simulink model "OvenMass"  (R2019b)
settings: Solver=VariableStepAuto  StartTime=0.0  StopTime=500  RelTol=1e-3
model workspace (MAT data in the model file):
  Stefan_Boltzmann_constant = 5.6704e-08
  air_density = 1.225
  air_heat_transfer_coefficient = 0.6
  air_volume_cubic_inch = 1152
  air_volume_cubic_meter = 0.0188778989947
  brick_count = 32
  brick_mass = 2.27
  emissivity_mass = 0.7
  mass_length = 0.1
  mass_mass = 1
  set_temperature = Simulink.Parameter
  set_temperature.Value = 1000
  set_temperature.DataType = 'auto'
  set_temperature.Dimensions = [1 1]
  wire_cross_sectional_area = Simulink.Parameter
  wire_cross_sectional_area.Value = 7.07e-06
  wire_cross_sectional_area.DataType = 'auto'
  wire_cross_sectional_area.Dimensions = [1 1]
  wire_length = Simulink.Parameter
  wire_length.Value = 2.44
  wire_length.DataType = 'auto'
  wire_length.Dimensions = [1 1]
  wire_outer_surface_area = 0.04363
  wire_resistivity = Simulink.Parameter
  wire_resistivity.Value = 0.000135
  wire_resistivity.DataType = 'auto'
  wire_resistivity.Dimensions = [1 1]
  wire_specific_heat = Simulink.Parameter
  wire_specific_heat.Value = 300
  wire_specific_heat.DataType = 'auto'
  wire_specific_heat.Dimensions = [1 1]
libraries: fl_lib x17, nesl_utility x5, ee_lib x4, simulink x2, eePwmGenerator x1
settings Model: SimulationMode=rapid-accelerator  Creator=Lenovo  LastModifiedBy=Lenovo
settings SolverCC: AlgebraicLoopSolver=LineSearch

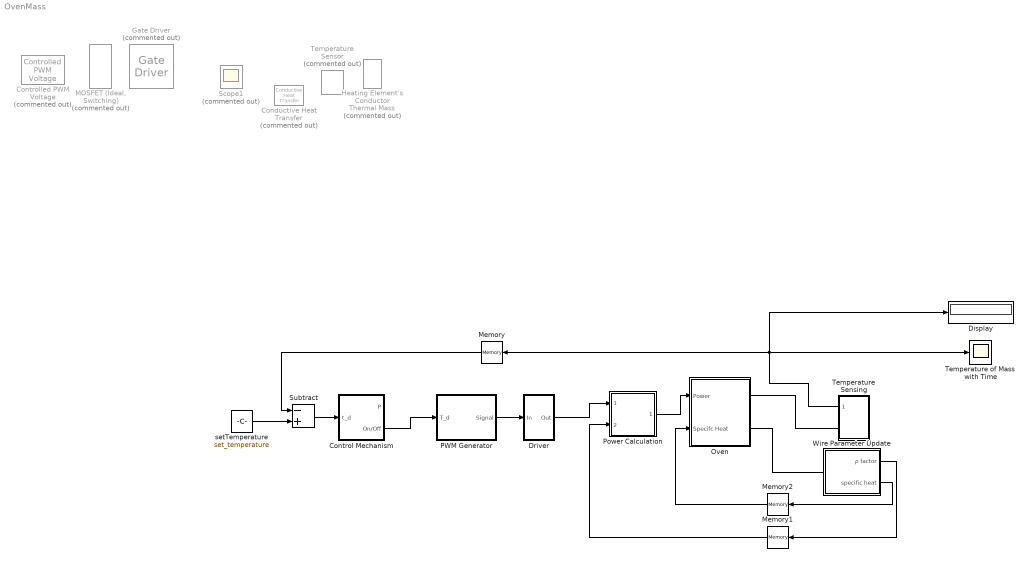
== system OvenMass ==
  Conductive Heat Transfer : fl_lib/Thermal/Thermal Elements/Conductive Heat Transfer  Commented=on  area=1e-4 m^2  thickness=0.1 m  th_cond=401 W/(m*K)  T_specify=off  T_priority=None  T=0 K  T_nominal_specify=off  T_nominal_unit=K  T_nominal_value=1  Q_specify=off  Q_priority=None  Q=0 W  Q_nominal_specify=off  Q_nominal_unit=W  Q_nominal_value=1
      settings: SourceProductName=Simscape
  Control Mechanism : Subsystem
  Controlled PWM Voltage : ee_lib/Integrated Circuits/Controlled PWM Voltage  Commented=on  F=1000 Hz  TD=0 s  pulse_width_offset=0 s  pulse_min=0 s  Vmin=0 V  Vmax=5 V  Vm=5 V  pwm_or_av=1  event_type=1  sample_time=1e-6 s  u_min=0  u_max=1
      settings: SourceProductName=Simscape Electrical  InternalSimscapePortConfiguration="{\"Bottom\":[],\"Left\":[{\"id\":\"u\",\"label\":\"u\",\"type\":\"input\"}],\"Right\":[{\"id\":\"p2\",\"label\":\"PWM\",\"type\":\"foundation.electrical.electrical\"},{\"id\":\"n2\",\"label\":\"REF\",\"type\":\"foundation.electrical.electrical\"}],\"Top\":[]}"
  Display : Display
      settings: Decimation=2
  Driver : Subsystem
  Gate Driver : ee_lib/Semiconductors & Converters/Gate Driver  Commented=on  vHigh=15 V  vLow=0 V  parameterization=1  rHigh=2 Ohm  rLow=2 Ohm  tRise=20 ns  tFall=20 ns  cLoad=10 nF  enable_faults=0  t_fault=1 s  fault_type=1  uHighValue=0.7  uLowValue=0.3  tHigh=50 ns  tLow=50 ns  ZonTime_specify=off  ZonTime_priority=None  ZonTime=0 s  ZoffTime_specify=off  ZoffTime_priority=None  ZoffTime=0 s  uHigh=2.0 V  uLow=0.8 V
      settings: SourceProductName=Simscape Electrical  SourceProductBaseCode=PS  InternalSimscapePortConfiguration="{\"Bottom\":[],\"Left\":[{\"id\":\"u\",\"label\":\"u\",\"type\":\"input\"}],\"Right\":[{\"id\":\"G\",\"label\":\"G\",\"type\":\"foundation.electrical.electrical\"},{\"id\":\"S\",\"label\":\"S\",\"type\":\"foundation.electrical.electrical\"}],\"Top\":[]}"
  Heating Element's Conductor : fl_lib/Thermal/Thermal Elements/Thermal Mass  Commented=on  mass=1 kg  sp_heat=780 J/kg/K  T_specify=off  T_priority=High  T=777 K  T_nominal_specify=off  T_nominal_unit=K  T_nominal_value=1  Q_specify=off  Q_priority=None  Q=0 W  Q_nominal_specify=off  Q_nominal_unit=W  Q_nominal_value=1
  "MOSFET (Ideal, Switching)" : ee_lib/Semiconductors & Converters/MOSFET (Ideal, Switching)  Commented=on  Rds=0.01 Ohm  Goff=1e-6 1/Ohm  Vth=2 V  diode_param=1  diode_Vf=0.8 V  diode_Ron=0.001 Ohm  diode_Goff=1e-5 1/Ohm  diode_C=50e-9 F  diode_iRM=-235 A  diode_iF=300 A  diode_idot=-50 A/us  diode_trr_param=1  diode_trr_factor=3  diode_trr=15 us  diode_Qrr=1500 s*uA  thermal_loss_option=2  Voff=300 V  Tau=1e-4 s  Tj=[298.15, 398.15] K  Iout_scalar=600 A  Eon_scalar=22.86e-3 J  Eoff_scalar=17.14e-3 J  Von_scalar=2.7 V  Iout_data=[0, 10, 50, 100, 200, 400, 600] A  Eon_data=[0, .29, 1.43, 2.86, 5.71, 13.14, 22.86; 0, .57, 2.63, 5.14, 10.29, 20.57, 30.29] * 1e-3 J  Eoff_data=[0, .21, 1.07, 2.14, 4.29, 9.86, 17.14; 0, .43, 1.97, 3.86, 7.71, 15.43, 22.71] * 1e-3 J  Von_data=[0, 1.1, 1.3, 1.45, 1.75, 2.25, 2.7; 0, 1, 1.15, 1.35, 1.7, 2.35, 3] V
      settings: SourceProductName=Simscape Electrical
  Memory : Memory  InitialCondition=set_temperature
  Memory1 : Memory  InitialCondition=1
  Memory2 : Memory  InitialCondition=0.46
  Oven : Subsystem
  PWM Generator : Subsystem
  Power Calculation : Subsystem
  Scope1 : Scope  Commented=on
  Subtract : Sum  Inputs=-+
  Temperature Sensing : Subsystem
  Temperature Sensor : fl_lib/Thermal/Thermal Sensors/Temperature Sensor  Commented=on
  Temperature of Mass with Time : Scope
  Wire Parameter Update : Subsystem
  setTemperature : Constant  Value=set_temperature
  wires:
  Subtract/1 -> Control Mechanism/1(t_d)
  PWM Generator/1(Signal) -> Driver/1(In)
  Temperature Sensing/1(T_mass) -> Display/1, Temperature of Mass with Time/1, Memory/1
  Memory1/1 -> Power Calculation/2(ρ Factor)
  Driver/1(Out) -> Power Calculation/1(Current)
  setTemperature/1 -> Subtract/2
  Memory/1 -> Subtract/1
  Power Calculation/1(Power) -> Oven/1(Power)
  Wire Parameter Update/1(ρ factor) -> Memory1/1
  Wire Parameter Update/2(specific heat) -> Memory2/1
  Memory2/1 -> Oven/2(Specifc Heat)
  Control Mechanism/2("On/Off ") -> PWM Generator/1(T_d)
  connections:
  Temperature Sensing/RConn1 -- Oven/RConn1
  Oven/RConn2 -- Wire Parameter Update/LConn1

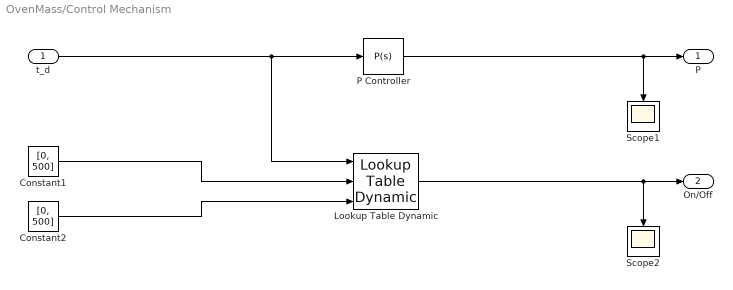
== system OvenMass/Control Mechanism ==
  t_d : Inport
  Constant1 : Constant  Value=[0, 500]
  Constant2 : Constant  Value=[0, 500]
  Lookup Table Dynamic : simulink/Lookup Tables/Lookup Table Dynamic  LookUpMeth=Use Input Above  OutDataType=fixdt('double')  OutScaling=[]  OutputDataTypeScalingMode=Specify via dialog  OutDataTypeStr=double  DoSatur=off
      settings: SourceProductName=Simulink
  P Controller : simulink/Continuous/PID Controller  Controller=P  Form=Parallel  TimeDomain=Continuous-time  SampleTime=-1  IntegratorMethod=Forward Euler  FilterMethod=Forward Euler  ControllerParametersSource=internal  P=10  I=0.5  D=0.5  UseFilter=on  N=100  TunerSelectOption=Frequency Response Based  InitialConditionSource=internal  InitialConditionForIntegrator=0  InitialConditionForFilter=0  DifferentiatorICPrevScaledInput=0  ExternalReset=none  TrackingMode=off  Kt=1  LimitOutput=off  UpperSaturationLimit=inf  LowerSaturationLimit=-inf  LinearizeAsGain=on  AntiWindupMode=none  Kb=1  POutMin=[]  POutMax=[]  IOutMin=[]  IOutMax=[]  DOutMin=[]  DOutMax=[]  NOutMin=[]  NOutMax=[]  SumOutMin=[]  SumOutMax=[]  SaturationOutMin=[]  SaturationOutMax=[]  PParamMin=[]  PParamMax=[]  IParamMin=[]  IParamMax=[]  DParamMin=[]  DParamMax=[]  NParamMin=[]  NParamMax=[]  KbParamMin=[]  KbParamMax=[]  KtParamMin=[]  KtParamMax=[]  KbOutMin=[]  KbOutMax=[]  KtOutMin=[]  KtOutMax=[]  IntegratorOutMin=[]  IntegratorOutMax=[]  FilterOutMin=[]  FilterOutMax=[]  SumI1OutMin=[]  SumI1OutMax=[]  SumI2OutMin=[]  SumI2OutMax=[]  SumI3OutMin=[]  SumI3OutMax=[]  SumI4OutMin=[]  SumI4OutMax=[]  SumDOutMin=[]  SumDOutMax=[]  DifferentiatorOutMin=[]  DifferentiatorOutMax=[]  FilterDiffOutCoefMin=[]  FilterDiffOutCoefMax=[]  ReciprocalOutMin=[]  ReciprocalOutMax=[]  SumDenOutMin=[]  SumDenOutMax=[]  SumNumOutMin=[]  SumNumOutMax=[]  DivideOutMin=[]  DivideOutMax=[]  IntegratorContinuousStateAttributes=''  IntegratorStateMustResolveToSignalObject=off  IntegratorRTWStateStorageClass=Auto  FilterContinuousStateAttributes=''  FilterStateMustResolveToSignalObject=off  FilterRTWStateStorageClass=Auto  ParallelPVariant=InternalParameters  IdealPVariant=Disabled  IVariant=Disabled  DVariant=Disabled  IntegratorVariant=Disabled  SatVariant=Disabled  AWVariant=Disabled  PCopyVariant=Disabled  TRVariant=Disabled  FdbkBlocksVariant=Forward  IdealPFdbkVariant=Disabled  SatFdbkVariant=Disabled  DerivativeFilterVariant=Disabled  NVariant=Disabled  NCopyVariant=Disabled_SignalSpec  FilterICVariant=Disabled  IntegratorICVariant=Disabled  ExternalResetVariant=Disabled  TRSumVariant=Passthrough  SumFdbkVariant=Disabled  SumVariant=Passthrough_P
  Scope1 : Scope
  Scope2 : Scope
  P : Outport
  "On/Off " : Outport  Port=2
  wires:
  Constant1/1 -> Lookup Table Dynamic/2
  Lookup Table Dynamic/1 -> "On/Off "/1, Scope2/1
  Constant2/1 -> Lookup Table Dynamic/3
  P Controller/1 -> P/1, Scope1/1
  t_d/1 -> P Controller/1, Lookup Table Dynamic/1

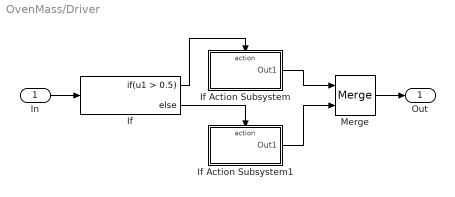
== system OvenMass/Driver ==
  In : Inport
  If : If  IfExpression=u1 > 0.5
  If Action Subsystem : Subsystem  TreatAsAtomicUnit=on
  If Action Subsystem1 : Subsystem  TreatAsAtomicUnit=on
  Merge : Merge
  Out : Outport
  wires:
  If/1 -> If Action Subsystem/Action
  If/2 -> If Action Subsystem1/Action
  In/1 -> If/1
  If Action Subsystem1/1(Out1) -> Merge/2
  If Action Subsystem/1(Out1) -> Merge/1
  Merge/1 -> Out/1

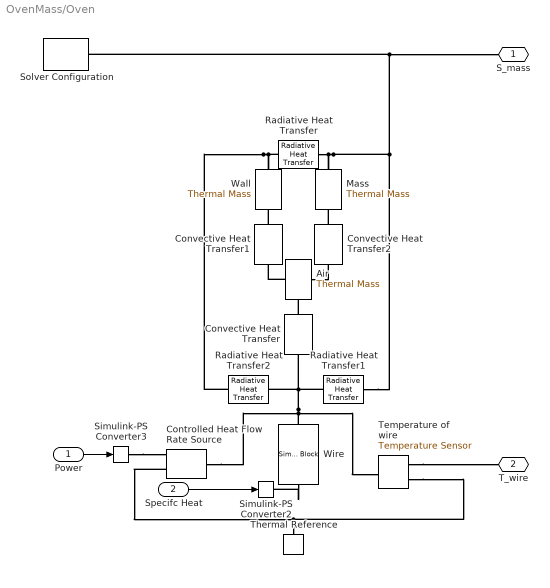
== system OvenMass/Oven ==
  Power : Inport
  Specifc Heat : Inport  Port=2
  Air : fl_lib/Thermal/Thermal Elements/Thermal Mass  mass=air_volume_cubic_meter kg  sp_heat=993 J/kg/K  T_specify=off  T_priority=High  T=300 K  T_nominal_specify=off  T_nominal_unit=K  T_nominal_value=1  Q_specify=off  Q_priority=None  Q=0 W  Q_nominal_specify=off  Q_nominal_unit=W  Q_nominal_value=1
  Controlled Heat Flow Rate Source : fl_lib/Thermal/Thermal Sources/Controlled Heat Flow Rate Source
      settings: SourceProductName=Simscape
  Convective Heat Transfer : fl_lib/Thermal/Thermal Elements/Convective Heat Transfer  area=wire_outer_surface_area m^2  heat_tr_coeff=air_heat_transfer_coefficient W/(m^2 * K)  T_specify=off  T_priority=None  T=0 K  T_nominal_specify=off  T_nominal_unit=K  T_nominal_value=1  Q_specify=off  Q_priority=None  Q=0 W  Q_nominal_specify=off  Q_nominal_unit=W  Q_nominal_value=1
  Convective Heat Transfer1 : fl_lib/Thermal/Thermal Elements/Convective Heat Transfer  area=3 * 8 * 2.25 * 4 * 2 in^2  heat_tr_coeff=air_heat_transfer_coefficient W/(m^2 * K)  T_specify=off  T_priority=None  T=0 K  T_nominal_specify=off  T_nominal_unit=K  T_nominal_value=1  Q_specify=off  Q_priority=None  Q=0 W  Q_nominal_specify=off  Q_nominal_unit=W  Q_nominal_value=1
  Convective Heat Transfer2 : fl_lib/Thermal/Thermal Elements/Convective Heat Transfer  area=5 * mass_length * mass_length m^2  heat_tr_coeff=air_heat_transfer_coefficient W/(m^2 * K)  T_specify=off  T_priority=None  T=0 K  T_nominal_specify=off  T_nominal_unit=K  T_nominal_value=1  Q_specify=off  Q_priority=None  Q=0 W  Q_nominal_specify=off  Q_nominal_unit=W  Q_nominal_value=1
  Mass : fl_lib/Thermal/Thermal Elements/Thermal Mass  mass=mass_mass kg  sp_heat=1420 J/kg/K  T_specify=off  T_priority=High  T=777 K  T_nominal_specify=off  T_nominal_unit=K  T_nominal_value=1  Q_specify=off  Q_priority=None  Q=0 W  Q_nominal_specify=off  Q_nominal_unit=W  Q_nominal_value=1
  Radiative Heat Transfer : fl_lib/Thermal/Thermal Elements/Radiative Heat Transfer  area=5 * mass_length * mass_length m^2  rad_tr_coeff=emissivity_mass * Stefan_Boltzmann_constant W/(m^2*K^4)  T_specify=off  T_priority=None  T=0 K  T_nominal_specify=off  T_nominal_unit=K  T_nominal_value=1  Q_specify=off  Q_priority=None  Q=0 W  Q_nominal_specify=off  Q_nominal_unit=W  Q_nominal_value=1
      settings: SourceProductName=Simscape  SourceProductBaseCode=SS  InternalSimscapePortConfiguration="{\"Bottom\":[],\"Left\":[{\"id\":\"A\",\"label\":\"A\",\"type\":\"foundation.thermal.thermal\"}],\"Right\":[{\"id\":\"B\",\"label\":\"B\",\"type\":\"foundation.thermal.thermal\"}],\"Top\":[]}"
  Radiative Heat Transfer1 : fl_lib/Thermal/Thermal Elements/Radiative Heat Transfer  area=wire_outer_surface_area m^2  rad_tr_coeff=(2.178e-9)/wire_outer_surface_area W/(m^2*K^4)  T_specify=off  T_priority=None  T=0 K  T_nominal_specify=off  T_nominal_unit=K  T_nominal_value=1  Q_specify=off  Q_priority=None  Q=0 W  Q_nominal_specify=off  Q_nominal_unit=W  Q_nominal_value=1
      settings: SourceProductName=Simscape  SourceProductBaseCode=SS  InternalSimscapePortConfiguration="{\"Bottom\":[],\"Left\":[{\"id\":\"A\",\"label\":\"A\",\"type\":\"foundation.thermal.thermal\"}],\"Right\":[{\"id\":\"B\",\"label\":\"B\",\"type\":\"foundation.thermal.thermal\"}],\"Top\":[]}"
  Radiative Heat Transfer2 : fl_lib/Thermal/Thermal Elements/Radiative Heat Transfer  area=wire_outer_surface_area m^2  rad_tr_coeff=(2.178e-9)/wire_outer_surface_area W/(m^2*K^4)  T_specify=off  T_priority=None  T=0 K  T_nominal_specify=off  T_nominal_unit=K  T_nominal_value=1  Q_specify=off  Q_priority=None  Q=0 W  Q_nominal_specify=off  Q_nominal_unit=W  Q_nominal_value=1
      settings: SourceProductName=Simscape  SourceProductBaseCode=SS  InternalSimscapePortConfiguration="{\"Bottom\":[],\"Left\":[{\"id\":\"A\",\"label\":\"A\",\"type\":\"foundation.thermal.thermal\"}],\"Right\":[{\"id\":\"B\",\"label\":\"B\",\"type\":\"foundation.thermal.thermal\"}],\"Top\":[]}"
  Simulink-PS Converter2 : nesl_utility/Simulink-PS Converter  PhysicalDomain=network_engine_domain  SubClassName=ps_input  LeftPortType=input  RightPortType=output  PseudoPeriodic=off  Frequencies=[]  NoiseDistribution=none  NoiseParameters=[]  Unit=1  AffineConversion=off  FilteringAndDerivatives=provide  SimscapeFilterOrder=1  InputFilterTimeConstant=0.001  UdotUserProvided=0
  Simulink-PS Converter3 : nesl_utility/Simulink-PS Converter  PhysicalDomain=network_engine_domain  SubClassName=ps_input  LeftPortType=input  RightPortType=output  PseudoPeriodic=off  Frequencies=[]  NoiseDistribution=none  NoiseParameters=[]  Unit=1  AffineConversion=off  FilteringAndDerivatives=provide  SimscapeFilterOrder=1  InputFilterTimeConstant=0.001  UdotUserProvided=0
  Solver Configuration : nesl_utility/Solver Configuration  PhysicalDomain=network_engine_domain  SubClassName=solver  LeftPortType=input  RightPortType=generic  Tones=[]  Harmonics=[]  SimulateNoise=off  Profile=off  UseLocalSampling=off  EnableSwitchedLinearOptims=on  FrequencyDomain=off  UseCCode=off  RelTol=0.001  AbsTol=1e-06  MinStep=1e-09  ToWorkspace=off  RevertToSquareIcSolve=off  NumHomotopyIterations=100  PhasorMode=off  PhasorModeNumHarmonics=1  DoDC=off  ResidualTolerance=1e-09  UseLocalSolver=off  LocalSolverChoice=NE_BACKWARD_EULER_ADVANCER  LocalSolverSampleTime=0.001  DoFixedCost=off  MaxNonlinIter=3  MaxModeIter=2  LinearAlgebra=auto  EquationFormulation=NE_TIME_EF  DelaysMemoryBudget=1024  AutomaticFiltering=on  FilteringTimeConstant=0.001  PartitionStorageMethod=AS_NEEDED  PartitionMemoryBudget=1024  PartitionMethod=ROBUST
  Temperature of wire : fl_lib/Thermal/Thermal Sensors/Temperature Sensor
  Thermal Reference : fl_lib/Thermal/Thermal Elements/Thermal Reference
  Wall : fl_lib/Thermal/Thermal Elements/Thermal Mass  mass=brick_mass * brick_count kg  sp_heat=800 J/kg/K  T_specify=off  T_priority=High  T=300 K  T_nominal_specify=off  T_nominal_unit=K  T_nominal_value=1  Q_specify=off  Q_priority=None  Q=0 W  Q_nominal_specify=off  Q_nominal_unit=W  Q_nominal_value=1
  Wire : SimscapeComponentBlock  SourceFile=mass  ComponentPath=mass  ComponentVariants=mass  ComponentVariantNames=mass  ClassName=mass  SchemaVersion=1  mass=0.06326 kg  T_specify=off  T_priority=High  T=300 K  T_nominal_specify=off  T_nominal_unit=K  T_nominal_value=1  Q_specify=off  Q_priority=None  Q=0 W  Q_nominal_specify=off  Q_nominal_unit=W  Q_nominal_value=1
      settings: CopyFcn=simscape.engine.sli.internal.componentblockcallback(gcbh,'COPY')  PreCopyFcn=simscape.engine.sli.internal.componentblockcallback(gcbh,'PRECOPY')  PreDeleteFcn=simscape.engine.sli.internal.componentblockcallback(gcbh,'PREDELETE')  InternalSimscapePortConfiguration="{\"Bottom\":[],\"Left\":[{\"id\":\"M\",\"label\":\"\",\"type\":\"foundation.thermal.thermal\"}],\"Right\":[{\"id\":\"sp_heat\",\"label\":\"Specific heat\",\"type\":\"input\"}],\"Top\":[]}"
      mask Type: Thermal Mass
  S_mass : PMIOPort  Side=Right
  T_wire : PMIOPort  Port=2  Side=Right
  wires:
  Power/1 -> Simulink-PS Converter3/1
  Specifc Heat/1 -> Simulink-PS Converter2/1
  connections:
  Convective Heat Transfer/RConn1 -- Convective Heat Transfer2/LConn1 -- Air/LConn1 -- Convective Heat Transfer1/LConn1
  Convective Heat Transfer1/RConn1 -- Radiative Heat Transfer2/RConn1 -- Radiative Heat Transfer/LConn1 -- Wall/LConn1
  Temperature of wire/RConn2 -- T_wire/RConn1
  Temperature of wire/RConn1 -- Controlled Heat Flow Rate Source/RConn2 -- Thermal Reference/LConn1
  Radiative Heat Transfer1/LConn1 -- Wire/LConn1 -- Controlled Heat Flow Rate Source/LConn1 -- Temperature of wire/LConn1 -- Radiative Heat Transfer2/LConn1 -- Convective Heat Transfer/LConn1
  Simulink-PS Converter3/RConn1 -- Controlled Heat Flow Rate Source/RConn1
  Wire/RConn1 -- Simulink-PS Converter2/RConn1
  Convective Heat Transfer2/RConn1 -- Radiative Heat Transfer1/RConn1 -- Solver Configuration/RConn1 -- S_mass/RConn1 -- Radiative Heat Transfer/RConn1 -- Mass/LConn1

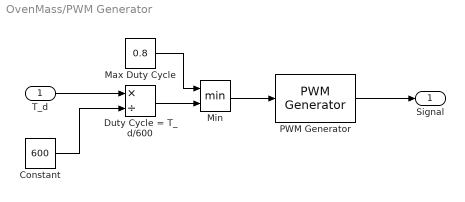
== system OvenMass/PWM Generator ==
  T_d : Inport
  Constant : Constant  Value=600
  Duty Cycle = T_d/600 : Product  Inputs=*/
  Max Duty Cycle : Constant  Value=0.8
  Min : MinMax  Inputs=2
  PWM Generator : eePwmGenerator/PWM Generator  CarrCount=Up  Tper=1/50  Ts=0
      settings: SourceProductName=Simscape Electrical
  Signal : Outport
  wires:
  PWM Generator/1 -> Signal/1
  Min/1 -> PWM Generator/1
  Constant/1 -> Duty Cycle = T_d/600/2
  T_d/1 -> Duty Cycle = T_d/600/1
  Duty Cycle = T_d/600/1 -> Min/2
  Max Duty Cycle/1 -> Min/1

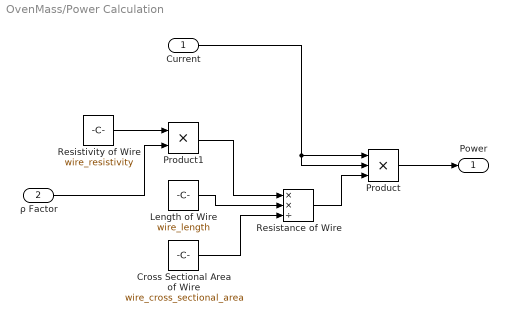
== system OvenMass/Power Calculation ==
  Current : Inport
  ρ Factor : Inport  Port=2
  Cross Sectional Area of Wire : Constant  Value=wire_cross_sectional_area
  Length of Wire : Constant  Value=wire_length
  Product : Product  Inputs=3
  Product1 : Product
  Resistance of Wire : Product  Inputs=**/
  Resistivity of Wire : Constant  Value=wire_resistivity
  Power : Outport
  wires:
  Length of Wire/1 -> Resistance of Wire/2
  Cross Sectional Area of Wire/1 -> Resistance of Wire/3
  Resistivity of Wire/1 -> Product1/1
  ρ Factor/1 -> Product1/2
  Product1/1 -> Resistance of Wire/1
  Product/1 -> Power/1
  Current/1 -> Product/1, Product/2
  Resistance of Wire/1 -> Product/3

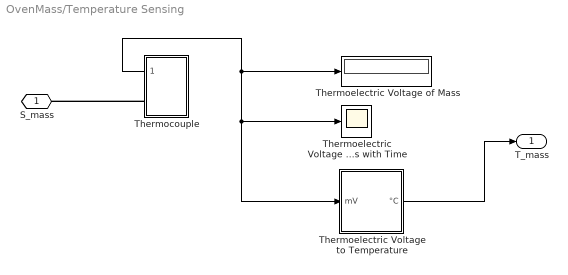
== system OvenMass/Temperature Sensing ==
  "Thermocouple " : Subsystem
  Thermoelectric Voltage of Mass : Display
  Thermoelectric Voltage of Mass with Time : Scope
  Thermoelectric Voltage to Temperature : Subsystem
  S_mass : PMIOPort  Side=Right
  T_mass : Outport
  wires:
  "Thermocouple "/1(Output) -> Thermoelectric Voltage to Temperature/1(mV), Thermoelectric Voltage of Mass with Time/1, Thermoelectric Voltage of Mass/1
  Thermoelectric Voltage to Temperature/1(°C) -> T_mass/1
  connections:
  "Thermocouple "/RConn1 -- S_mass/RConn1

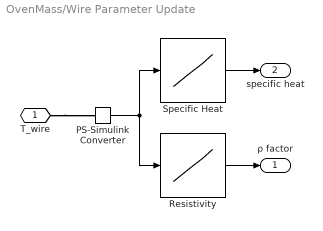
== system OvenMass/Wire Parameter Update ==
  PS-Simulink Converter : nesl_utility/PS-Simulink Converter  PhysicalDomain=network_engine_domain  SubClassName=ps_output  LeftPortType=input  RightPortType=output  PseudoPeriodic=off  Frequencies=[]  Unit=inherit  AffineConversion=off
  Resistivity : Lookup_n-D  NumberOfTableDimensions=1  BreakpointsForDimension1=[0,100,200,300,400,500,600,700,800,900,1000,1100,1200,1300]  Table=[1.00,1.00,1.01,1.01,1.02,1.03,1.04,1.05,1.06,1.07,1.07,1.07,1.08,1.08]  InterpMethod=Linear Lagrange  InternalRulePriority=Speed  RndMeth=Simplest  InputSameDT=on
  Specific Heat : Lookup_n-D  NumberOfTableDimensions=1  BreakpointsForDimension1=[20,200,400,600,800,1000,1200]  Table=[0.46,0.56,0.63,0.75,0.71,0.72,0.74]  InterpMethod=Linear Lagrange  InternalRulePriority=Speed  RndMeth=Simplest  InputSameDT=on
  T_wire : PMIOPort  Side=Left
  ρ factor : Outport
  specific heat : Outport  Port=2
  wires:
  Resistivity/1 -> ρ factor/1
  Specific Heat/1 -> specific heat/1
  PS-Simulink Converter/1 -> Resistivity/1, Specific Heat/1
  connections:
  T_wire/RConn1 -- PS-Simulink Converter/LConn1

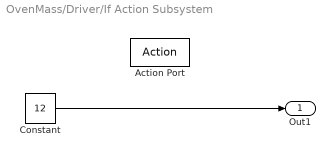
== system OvenMass/Driver/If Action Subsystem ==
  Action Port : ActionPort  ActionPortLabel=if(u1 > 0.5)
  Constant : Constant  Value=12
  Out1 : Outport
  wires:
  Constant/1 -> Out1/1

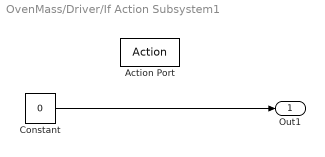
== system OvenMass/Driver/If Action Subsystem1 ==
  Action Port : ActionPort  ActionPortLabel=else
  Constant : Constant  Value=0
  Out1 : Outport
  wires:
  Constant/1 -> Out1/1

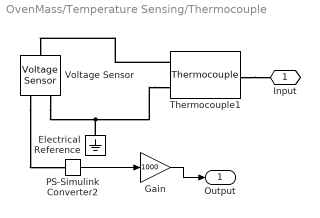
== system OvenMass/Temperature Sensing/Thermocouple  ==
  Electrical Reference : fl_lib/Electrical/Electrical Elements/Electrical Reference
  Gain : Gain  Gain=1000
  PS-Simulink Converter2 : nesl_utility/PS-Simulink Converter  PhysicalDomain=network_engine_domain  SubClassName=ps_output  LeftPortType=input  RightPortType=output  PseudoPeriodic=off  Frequencies=[]  Unit=inherit  AffineConversion=off
  Thermocouple1 : ee_lib/Sensors & Transducers/Thermocouple  thermocouple_type=2  Cvec=[-0.176004136860e-1, 0.389212049750e-1, 0.185587700320e-4, -0.994575928740e-7, 0.318409457190e-9, -0.560728448890e-12, 0.560750590590e-15, -0.320207200030e-18, 0.971511471520e-22,-0.121047212750e-25]  Avec=[0.118597600000, -0.118343200000e-3, 0.126968600000e3]  T0=0 degC  tc=1 s  K_d=1e-3 W/K  init_temp=25 degC
      settings: SourceProductName=Simscape Electrical  SourceProductBaseCode=PS  InternalSimscapePortConfiguration="{\"Bottom\":[],\"Left\":[{\"id\":\"p\",\"label\":\"+\",\"type\":\"foundation.electrical.electrical\"},{\"id\":\"n\",\"label\":\"-\",\"type\":\"foundation.electrical.electrical\"}],\"Right\":[{\"id\":\"A\",\"label\":\"A\",\"type\":\"foundation.thermal.thermal\"}],\"Top\":[]}"
  Voltage Sensor : fl_lib/Electrical/Electrical Sensors/Voltage Sensor
  "Input " : PMIOPort  Side=Right
  Output : Outport
  wires:
  PS-Simulink Converter2/1 -> Gain/1
  Gain/1 -> Output/1
  connections:
  Thermocouple1/LConn2 -- Voltage Sensor/RConn2 -- Electrical Reference/LConn1
  Voltage Sensor/RConn1 -- PS-Simulink Converter2/LConn1
  Thermocouple1/RConn1 -- "Input "/RConn1
  Thermocouple1/LConn1 -- Voltage Sensor/LConn1

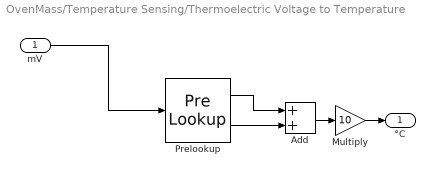
== system OvenMass/Temperature Sensing/Thermoelectric Voltage to Temperature ==
  mV : Inport
  Add : Sum
  Multiply : Gain  Gain=10
  Prelookup : PreLookup  BreakpointsData=[0.0, 0.397, 0.798, 1.203, 1.612, 2.023, 2.436, 2.851, 3.267, 3.682, 4.096, 4.509, 4.92, 5.328, 5.735, 6.138, 6.54, 6.941, 7.34, 7.739, 8.138, 8.539, 8.94, 9.343, 9.747, 10.153, 10.561, 10.971, 11.382, 11.795, 12.209, 12.624, 13.04, 13.457, 13.874, 14.293, 14.713, 15.133, 15.554, 15.975, 16.397, 16.82, 17.243, 17.667, 18.091, 18.516, 18.941, 19.366, 19.792, 20.218, 20.644, 21.071, 21.497, 21.924, 22.35, 22.776, 23.203, 23.629, 24.055, 24.48, 24.905, 25.33, 25.755, 26.179, 26.602, 27.025, 27.447, 27.869, 28.289, 28.71, 29.129, 29.548, 29.965, 30.382, 30.798, 31.213, 31.628, 32.041, 32.453, 32.865, 33.275, 33.685, 34.093, 34.501, 34.908, 35.313, 35.718, 36.121, 36.524, 36.925, 37.326, 37.725, 38.124, 38.522, 38.918, 39.314, 39.708, 40.101, 40.494, 40.885, 41.276, 41.665, 42.053, 42.44, 42.826, 43.211, 43.595, 43.978, 44.359, 44.74, 45.119, 45.497, 45.873, 46.249, 46.623, 46.995, 47.367, 47.737, 48.105, 48.473, 48.838, 49.202, 49.565, 49.926, 50.286, 50.644, 51.0, 51.355, 51.708, 52.06, 52.41, 52.759, 53.106, 53.451, 53.795, 54.138, 54.479, 54.819]  ExtrapMethod=Linear  DiagnosticForOutOfRangeInput=Warning
  °C : Outport
  wires:
  Multiply/1 -> °C/1
  mV/1 -> Prelookup/1
  Add/1 -> Multiply/1
  Prelookup/1 -> Add/1
  Prelookup/2 -> Add/2
